simulink model "MS_test"  (R2023b)
settings: Solver=VariableStepAuto  StartTime=0.0  StopTime=10.0  RelTol=1e-3
undefined symbols (not defined in the file): dt, x0
settings Model: Creator=kasek  LastModifiedBy=sekiguchi

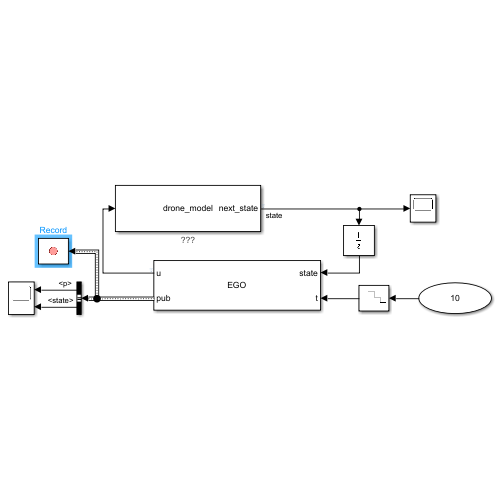
[thumbnail: Simulink's stored preview of the top-level diagram]
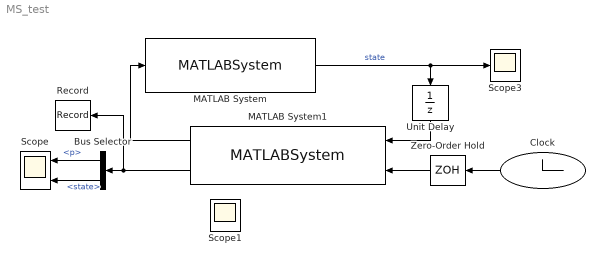
== system MS_test ==
  Bus Selector : BusSelector  OutputSignals=rresult.state.p,eresult.state
  Clock : Clock
  MATLAB System : MATLABSystem  System=drone_model  SimulateUsing=Code generation
      settings: AttributesFormatString=%<A>
      mask Type: drone_model
      mask Display:
      | disp('drone_model');
      | port_label('output',1,'next_state');
  MATLAB System1 : MATLABSystem  System=EGO  SimulateUsing=Code generation
      mask Type: EGO
      mask Display:
      | disp('EGO');
      | port_label('input',1,'state');
      | port_label('input',2,'t');
      | port_label('output',1,'u');
      | port_label('output',2,'pub');
  Record : Record  FileSettingsInternal="{\"entries\":[{\"content\":{\"excelSettings\":{\"content\":{},\"type\":\"Streamout.ExcelSettings\"}},\"type\":\"Streamout.FileSettingStorage\",\"uuid\":\"\"}],\"packageUris\":[\"http:\\/\\/schema.mathworks.com\\/mf0\\/streamout_blocks\\/R2020a\"],\"version\":\"1.0\"}"  SignalsInternal="{\"entries\":[{\"content\":{\"signals\":[{\"content\":{\"blockPath\":[],\"dimensions\":[1,1],\"domain\":\"\",\"hasChildren\":true,\"lineColor\":\"#0072bd\",\"port\":1,\"sid\":[\"\"],\"signalID\":1,\"signalName\":\"MATLAB System1:2\"},\"type\":\"RecordBlkView.Signal\",\"uuid\":\"\"},{\"content\":{\"blockPath\":[],\"dimensions\":[1],\"domain\":\"\",\"hasChildren\":true,\"lineColor\":\"#d95319\",\"parentID\":1,\"port\":1,\"sid\":[\"\"],\"signalID\":2,\"signalName\":\"rresult\"},\"type\":\"RecordBlkView.Signal\",\"uuid\":\"\"},{\"content\":{\"blockPath\":[],\"dimensions\":[1],\"domain\":\"\",\"hasChildren\":true,\"lineColor\":\"#edb120\",\"parentID\":2,\"port\":1,\"sid\":[\"\"],\"signalID\":3,\"signalName\":\"state\"},\"type\":\"RecordBlkView.Signal\",\"uuid\":\"\"},{\"content\":{\"blockPath\":[],\"dimensions\":[20,1],\"domain\":\"\",\"hasChildren\":true,\"lineColor\":\"#7e2f8e\",\"parentID\":3,\"port\":1,\"sid\":[\"\"],\"signalID\":4,\"signalName\":\"MATLAB System1:2.rresult.state.xd\"},\"type\":\"RecordBlkView.Signal\",\"uuid\":\"\"},{\"content\":{\"blockPath\":[],\"channel\":[1,1],\"dimensions\":[20,1],\"domain\":\"\",\"leafPath\":\"MATLAB System1:2.rresult.state.xd\",\"lineColor\":\"#77ac30\",\"parentID\":4,\"plots\":[ 1 ],\"port\":1,\"sid\":[\"\"],\"signalID\":5,\"signalName\":\"MATLAB System1:2.rresult.state.xd\"},\"type\":\"RecordBlkView.Signal\",\"uuid\":\"\"},{\"content\":{\"blockPath\":[],\"dimensions\":[3,1],\"domain\":\"\",\"hasChildren\":true,\"lineColor\":\"#4dbeee\",\"parentID\":3,\"port\":1,\"sid\":[\"\"],\"signalID\":6,\"signalName\":\"MATLAB System1:2.rresult.state.p\"},\"type\":\"RecordBlkView.Signal\",\"uuid\":\"\"},{\"content\":{\"blockPath\":[],\"channel\":[1,1],\"dimensions\":[3,1],\"domain\":\"\",\"leafPath\":\"MATLAB System1:2.rresult.state.p\",\"lineColor\":\"#a2142f\",\"parentID\":6,\"plots\":[ 1 ],\"port\":1,\"sid\":[\"\"],\"signalID\":7,\"signalName\":\"MATLAB System1:2.rresult.state.p\"},\"type\":\"RecordBlkView.Signal\",\"uuid\":\"\"},{\"content\":{\"blockPath\":[],\"dimensions\":[3,1],\"domain\":\"\",\"hasChildren\":true,\"lineColor\":\"#139fff\",\"parentID\":3,\"port\":1,\"sid\":[\"\"],\"signalID\":8,\"signalName\":\"MATLAB System1:2.rresult.state.v\"},\"type\":\"RecordBlkView.Signal\",\"uuid\":\"\"},{\"content\":{\"blockPath\":[],\"channel\":[1,1],\"dimensions\":[3,1],\"domain\":\"\",\"leafPath\":\"MATLAB System1:2.rresult.state.v\",\"lineColor\":\"#ff6929\",\"parentID\":8,\"plots\":[ 1 ],\"port\":1,\"sid\":[\"\"],\"signalID\":9,\"signalName\":\"MATLAB System1:2.rresult.state.v\"},\"type\":\"RecordBlkView.Signal\",\"uuid\":\"\"},{\"content\":{\"blockPath\":[],\"dimensions\":[3,1],\"domain\":\"\",\"hasChildren\":true,\"lineColor\":\"#b746ff\",\"parentID\":3,\"port\":1,\"sid\":[\"\"],\"signalID\":10,\"signalName\":\"MATLAB System1:2.rresult.state.q\"},\"type\":\"RecordBlkView.Signal\",\"uuid\":\"\"},{\"content\":{\"blockPath\":[],\"channel\":[1,1],\"dimensions\":[3,1],\"domain\":\"\",\"leafPath\":\"MATLAB System1:2.rresult.state.q\",\"lineColor\":\"#64d413\",\"parentID\":10,\"plots\":[ 1 ],\"port\":1,\"sid\":[\"\"],\"signalID\":11,\"signalName\":\"MATLAB System1:2.rresult.state.q\"},\"type\":\"RecordBlkView.Signal\",\"uuid\":\"\"},{\"content\":{\"blockPath\":[],\"dimensions\":[1],\"domain\":\"\",\"hasChildren\":true,\"lineColor\":\"#ff13a6\",\"parentID\":1,\"port\":1,\"sid\":[\"\"],\"signalID\":12,\"signalName\":\"eresult\"},\"type\":\"RecordBlkView.Signal\",\"uuid\":\"\"},{\"content\":{\"blockPath\":[],\"dimensions\":[12,1],\"domain\":\"\",\"hasChildren\":true,\"lineColor\":\"#fe330a\",\"parentID\":12,\"port\":1,\"sid\":[\"\"],\"signalID\":13,\"signalName\":\"MATLAB System1:2.eresult.state\"},\"type\":\"RecordBlkView.Signal\",\"uuid\":\"\"},{\"content\":{\"blockPath\":[],\"channel\":[1,1],\"dimensions\":[12,1],\"domain\":\"\",\"leafPath\":\"MATLAB System1:2.eresult.state\",\"lineColor\":\"#22b573\",\"parentID\":13,\"plots\":[ 1 ],\"port\":1,\"sid\":[\"\"],\"signalID\":14,\"signalName\":\"MATLAB System1:2.eresult.state\"},\"type\":\"RecordBlkView.Signal\",\"uuid\":\"\"},{\"content\":{\"blockPath\":[],\"dimensions\":[12,12],\"domain\":\"\",\"hasChildren\":true,\"lineColor\":\"#0072bd\",\"parentID\":12,\"port\":1,\"sid\":[\"\"],\"signalID\":15,\"signalName\":\"MATLAB System1:2.eresult.P\"},\"type\":\"RecordBlkView.Signal\",\"uuid\":\"\"},{\"content\":{\"blockPath\":[],\"channel\":[1,1],\"dimensions\":[12,12],\"domain\":\"\",\"leafPath\":\"MATLAB System1:2.eresult.P\",\"lineColor\":\"#d95319\",\"parentID\":15,\"plots\":[ 1 ],\"port\":1,\"sid\":[\"\"],\"signalID\":16,\"signalName\":\"MATLAB System1:2.eresult.P\"},\"type\":\"RecordBlkView.Signal\",\"uuid\":\"\"},{\"content\":{\"blockPath\":[],\"dimensions\":[1],\"domain\":\"\",\"hasChildren\":true,\"lineColor\":\"#edb120\",\"parentID\":1,\"port\":1,\"sid\":[\"\"],\"signalID\":17,\"signalName\":\"cresult\"},\"type\":\"RecordBlkView.Signal\",\"uuid\":\"\"},{\"content\":{\"blockPath\":[],\"dimensions\":[4,1],\"domain\":\"\",\"hasChildren\":true,\"lineColor\":\"#7e2f8e\",\"parentID\":17,\"port\":1,\"sid\":[\"\"],\"signalID\":18,\"signalName\":\"MATLAB System1:2.cresult.input\"},\"type\":\"RecordBlkView.Signal\",\"uuid\":\"\"},{\"content\":{\"blockPath\":[],\"channel\":[1,1],\"dimensions\":[4,1],\"domain\":\"\",\"leafPath\":\"MATLAB System1:2.cresult.input\",\"lineColor\":\"#77ac30\",\"parentID\":18,\"plots\":[ 1 ],\"port\":1,\"sid\":[\"\"],\"signalID\":19,\"signalName\":\"MATLAB System1:2.cresult.input\"},\"type\":\"RecordBlkView.Signal\",\"uuid\":\"\"},{\"content\":{\"blockPath\":[],\"channel\":[2,1],\"dimensions\":[3,1],\"domain\":\"\",\"leafPath\":\"MATLAB System1:2.rresult.state.p\",\"lineColor\":\"#ff6929\",\"parentID\":6,\"plots\":[ 1 ],\"port\":1,\"sid\":[\"\"],\"signalID\":20,\"signalName\":\"MATLAB System1:2.rresult.state.p\"},\"type\":\"RecordBlkView.Signal\",\"uuid\":\"\"},{\"content\":{\"blockPath\":[],\"channel\":[3,1],\"dimensions\":[3,1],\"domain\":\"\",\"leafPath\":\"MATLAB System1:2.rresult.state.p\",\"lineColor\":\"#b746ff\",\"parentID\":6,\"plots\":[ 1 ],\"port\":1,\"sid\":[\"\"],\"signalID\":21,\"signalName\":\"MATLAB System1:2.rresult.state.p\"},\"type\":\"RecordBlkView.Signal\",\"uuid\":\"\"},{\"content\":{\"blockPath\":[],\"channel\":[2,1],\"dimensions\":[3,1],\"domain\":\"\",\"leafPath\":\"MATLAB System1:2.rresult.state.v\",\"lineColor\":\"#64d413\",\"parentID\":8,\"plots\":[ 1 ],\"port\":1,\"sid\":[\"\"],\"signalID\":22,\"signalName\":\"MATLAB System1:2.rresult.state.v\"},\"type\":\"RecordBlkView.Signal\",\"uuid\":\"\"},{\"content\":{\"blockPath\":[],\"channel\":[3,1],\"dimensions\":[3,1],\"domain\":\"\",\"leafPath\":\"MATLAB System1:2.rresult.state.v\",\"lineColor\":\"#ff13a6\",\"parentID\":8,\"plots\":[ 1 ],\"port\":1,\"sid\":[\"\"],\"signalID\":23,\"signalName\":\"MATLAB System1:2.rresult.state.v\"},\"type\":\"RecordBlkView.Signal\",\"uuid\":\"\"},{\"content\":{\"blockPath\":[],\"channel\":[2,1],\"dimensions\":[3,1],\"domain\":\"\",\"leafPath\":\"MATLAB System1:2.rresult.state.q\",\"lineColor\":\"#fe330a\",\"parentID\":10,\"plots\":[ 1 ],\"port\":1,\"sid\":[\"\"],\"signalID\":24,\"signalName\":\"MATLAB System1:2.rresult.state.q\"},\"type\":\"RecordBlkView.Signal\",\"uuid\":\"\"},{\"content\":{\"blockPath\":[],\"channel\":[3,1],\"dimensions\":[3,1],\"domain\":\"\",\"leafPath\":\"MATLAB System1:2.rresult.state.q\",\"lineColor\":\"#22b573\",\"parentID\":10,\"plots\":[ 1 ],\"port\":1,\"sid\":[\"\"],\"signalID\":25,\"signalName\":\"MATLAB System1:2.rresult.state.q\"},\"type\":\"RecordBlkView.Signal\",\"uuid\":\"\"},{\"content\":{\"blockPath\":[],\"channel\":[2,1],\"dimensions\":[4,1],\"domain\":\"\",\"leafPath\":\"MATLAB System1:2.cresult.input\",\"lineColor\":\"#0072bd\",\"parentID\":18,\"plots\":[ 1 ],\"port\":1,\"sid\":[\"\"],\"signalID\":26,\"signalName\":\"MATLAB System1:2.cresult.input\"},\"type\":\"RecordBlkView.Signal\",\"uuid\":\"\"},{\"content\":{\"blockPath\":[],\"channel\":[3,1],\"dimensions\":[4,1],\"domain\":\"\",\"leafPath\":\"MATLAB System1:2.cresult.input\",\"lineColor\":\"#d95319\",\"parentID\":18,\"plots\":[ 1 ],\"port\":1,\"sid\":[\"\"],\"signalID\":27,\"signalName\":\"MATLAB System1:2.cresult.input\"},\"type\":\"RecordBlkView.Signal\",\"uuid\":\"\"},{\"content\":{\"blockPath\":[],\"channel\":[4,1],\"dimensions\":[4,1],\"domain\":\"\",\"leafPath\":\"MATLAB System1:2.cresult.input\",\"lineColor\":\"#edb120\",\"parentID\":18,\"plots\":[ 1 ],\"port\":1,\"sid\":[\"\"],\"signalID\":28,\"signalName\":\"MATLAB System1:2.cresult.input\"},\"type\":\"RecordBlkView.Signal\",\"uuid\":\"\"}]},\"type\":\"RecordBlkView.InputSignals\",\"uuid\":\"\"}],\"packageUris\":[\"http:\\/\\/schema.mathworks.com\\/mf0\\/streamout_blocks\\/R2020a\"],\"version\":\"1.0\"}"  VisualizationBindings="{\"sparklinesplugin\":{\"info\":[{\"bindingParametersList\":[],\"subplotID\":1}]}}"
  Scope : Scope  NumInputPorts=2
  Scope3 : Scope
  Unit Delay : UnitDelay  InitialCondition=x0  SampleTime=dt  HasFrameUpgradeWarning=on
  Zero-Order Hold : ZeroOrderHold  SampleTime=dt
  Scope1 : Scope
  wires:
  MATLAB System/1 -> Scope3/1, Unit Delay/1  "state"
  Clock/1 -> Zero-Order Hold/1
  Zero-Order Hold/1 -> MATLAB System1/2
  MATLAB System1/1 -> MATLAB System/1
  Unit Delay/1 -> MATLAB System1/1
  Bus Selector/1 -> Scope/1  "<p>"
  Bus Selector/2 -> Scope/2  "<state>"
  MATLAB System1/2 -> Record/1, Bus Selector/1
